simulink model "EcuAppM_StateMachine"  (R2022b)
settings: Solver=FixedStepDiscrete  StartTime=0  StopTime=50  FixedStep=1  RelTol=1e-3  EnableMultiTasking=on
values from neighbouring files (symbols this model uses):
  ECUAPPM_MAX_WAKEUP_SOURCES = mpt.Parameter    [EcuAppM_StateMachine_Param.m]    (also in EcuAppM_StateMachine_Param_For_Safety_Context.m)
  ECUAPPM_VALUE_ZERO = mpt.Parameter    [EcuAppM_StateMachine_Param.m]    (also in EcuAppM_StateMachine_Param_For_Safety_Context.m)
  EcuAppM_WakeupSourcesData = mpt.Parameter    [EcuAppM_StateMachine_Param.m]    (also in EcuAppM_StateMachine_Param_For_Safety_Context.m)
libraries: simulink x3
(part 1 of 2)
settings Model: Creator=CINISSAN  LastModifiedBy=akappa
settings SolverCC: AlgebraicLoopSolver=TrustRegion
settings DataIOCC: MaxDataPoints=1000000  SaveOutput=off  InspectSignalLogs=on  ReturnWorkspaceOutputs=off
settings OptimizationCC: DefaultParameterBehavior=Inlined  UseSpecifiedMinMax=on  PassReuseOutputArgsAs=Individual arguments  RollThreshold=2  ZeroExternalMemoryAtStartup=off  LifeSpan=1  MaxStackSize=750  OptimizationLevel=level1  EfficientTunableParamExpr=on
settings DebuggingCC: UnconnectedInputMsg=warning  UnconnectedOutputMsg=warning  UnconnectedLineMsg=warning  AllowSymbolicDim=off  SFUnexpectedBacktrackingDiag=warning  SFNoUnconditionalDefaultTransitionDiag=warning  SFExecutionAtInitializationDiag=none  SFMachineParentedDataDiag=warning  ArithmeticOperatorsInVariantConditions=warning
settings HardwareCC: ProdLongLongMode=on
settings ModelReferenceCC: EnableRefExpFcnMdlSchedulingChecks=on
settings SFSimCC: SimCustomHeaderCode="#include \"EcuAppMExt.h\""  SimUserSources=EcuAppMExt.c  SimUseLocalCustomCode=off  SimGenImportedTypeDefs=on  MATLABDynamicMemAlloc=off  CustomCodeUndefinedFunction=UseInterfaceOnly
settings RTWCC: Description=Embedded Coder  SystemTargetFile=ert.tlc  GenCodeOnly=on  TemplateMakefile=ert_default_tmf  GenerateReport=on  RetainRTWFile=on  RTWUseLocalCustomCode=off  CustomHeaderCode="#include \"EcuAppM_CmdProcessing.h\""  IncludeHyperlinkInReport=on  LaunchReport=on  PortableWordSizes=on  GenerateTraceInfo=on  GenerateTraceReport=on  GenerateTraceReportSl=on  GenerateTraceReportSf=on  GenerateTraceReportEml=on  GenerateCodeReplacementReport=on
settings CodeAppCC: IgnoreCustomStorageClasses=off  MaxIdLength=250  SimulinkBlockComments=off
settings ERTTargetCC: MultiwordLength=2048  GenerateSampleERTMain=on  SuppressErrorStatus=on  ParenthesesLevel=Maximum  CastingMode=Standards  InlinedParameterPlacement=NonHierarchical  ERTCustomFileTemplate=example_file_process.tlc  ERTFilePackagingFormat=CompactWithDataFile
settings ConfigComp: CovEnable=on  RecordCoverage=on  CovMetricSettings=dcmtw  CovHTMLOptions=-sRT=1 -sVT=0 -aTS=1 -agT=1 -bRG=1 -bTC=1 -hTR=0 -nFC=0 -nFD=1 -scm=1 -bcm=1 -xEv=1 -xEM=1 -req=1  CovSaveCumulativeToWorkspaceVar=on  CovCumulativeReport=on  CovModelRefEnable=on

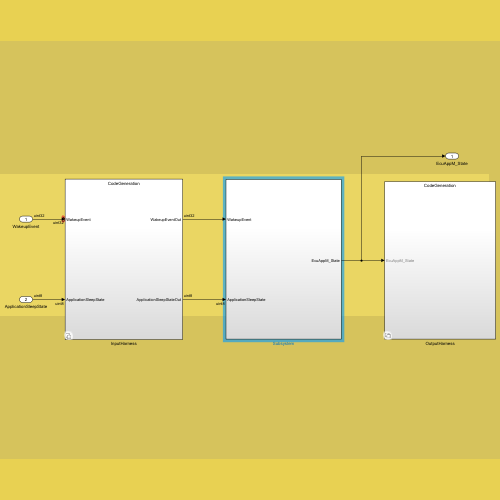
[thumbnail: Simulink's stored preview of the top-level diagram]
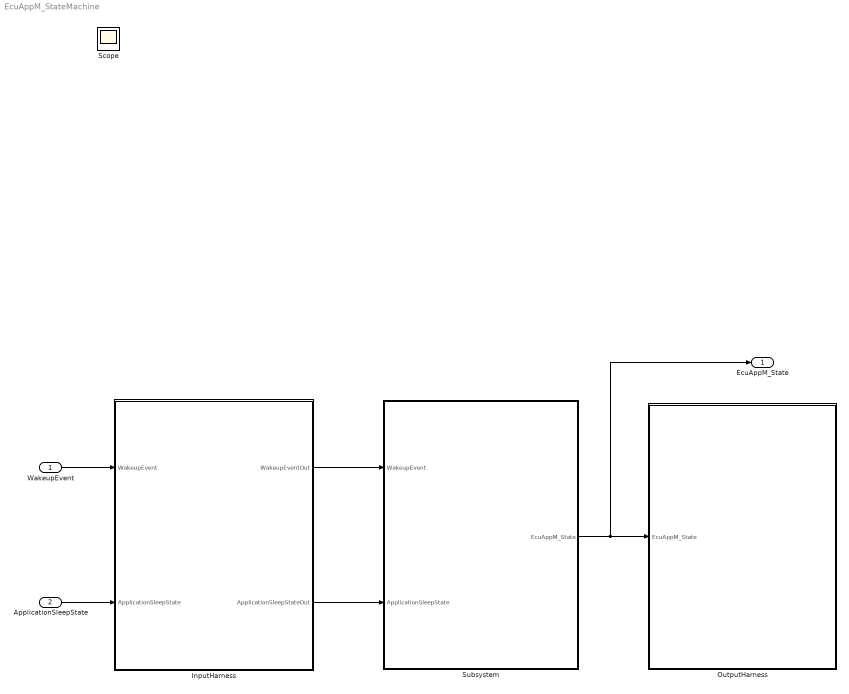
== system EcuAppM_StateMachine ==
  WakeupEvent : Inport  OutDataTypeStr=uint32
  ApplicationSleepState : Inport  Port=2  OutDataTypeStr=uint8
  InputHarness : Subsystem  Variant=on
  OutputHarness : Subsystem  Variant=on
  Subsystem : Subsystem
  EcuAppM_State : Outport  VectorParamsAs1DForOutWhenUnconnected=off
  Scope : Scope
  wires:
  ApplicationSleepState/1 -> InputHarness/2(ApplicationSleepState)
  InputHarness/1(WakeupEventOut) -> Subsystem/1(WakeupEvent)
  InputHarness/2(ApplicationSleepStateOut) -> Subsystem/2(ApplicationSleepState)
  Subsystem/1(EcuAppM_State) -> EcuAppM_State/1, OutputHarness/1(EcuAppM_State)
  WakeupEvent/1 -> InputHarness/1(WakeupEvent)

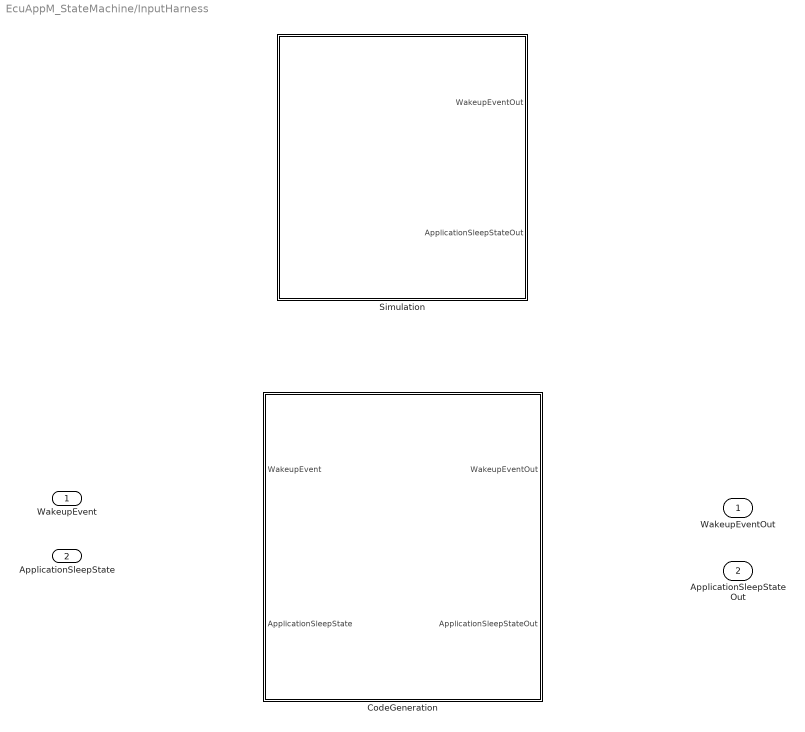
== system EcuAppM_StateMachine/InputHarness ==
  WakeupEvent : Inport  OutDataTypeStr=uint32
  ApplicationSleepState : Inport  Port=2  OutDataTypeStr=uint8
  CodeGeneration : Subsystem  VariantControl=CODEGENERATION
  Simulation : Subsystem  VariantControl=SIMULATION
  WakeupEventOut : Outport  OutDataTypeStr=uint32  PortDimensions=1  VectorParamsAs1DForOutWhenUnconnected=off
  ApplicationSleepStateOut : Outport  Port=2  OutDataTypeStr=uint8  PortDimensions=1  VectorParamsAs1DForOutWhenUnconnected=off

== system EcuAppM_StateMachine/OutputHarness ==
  EcuAppM_State : Inport
  CodeGeneration : Subsystem  VariantControl=CODEGENERATION
  Simulation : Subsystem  VariantControl=SIMULATION

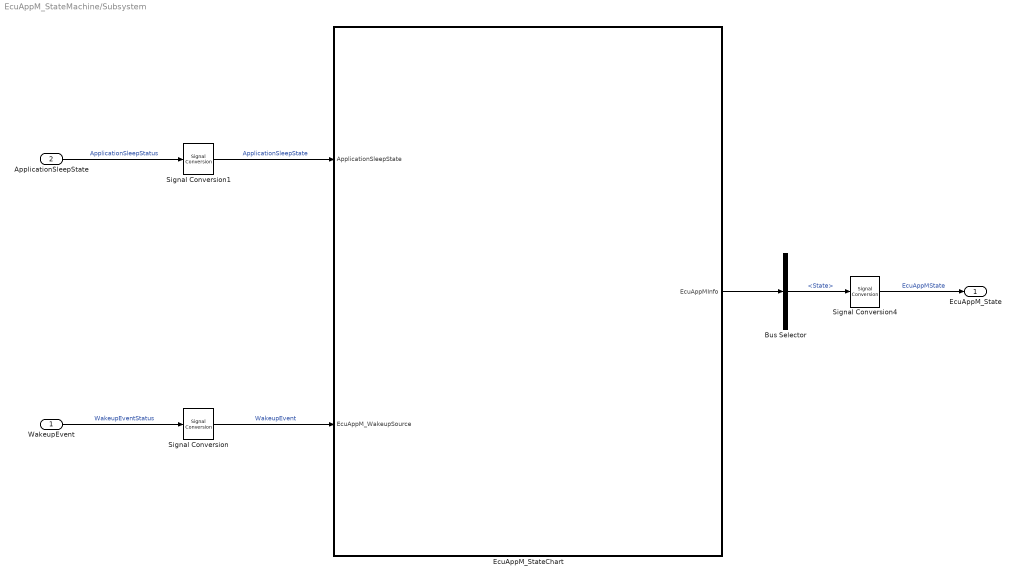
== system EcuAppM_StateMachine/Subsystem ==
  WakeupEvent : Inport  OutDataTypeStr=uint32
  ApplicationSleepState : Inport  Port=2  OutDataTypeStr=uint8
  Bus Selector : BusSelector  OutputSignals=State
  EcuAppM_StateChart : Stateflow chart  TreatAsAtomicUnit=on  RTWFcnName=EcuAppM_StateChart
      settings: RTWSystemCode=Nonreusable function  RTWFcnNameOpts=User specified
  Signal Conversion : SignalConversion  OverrideOpt=off
  Signal Conversion1 : SignalConversion  OverrideOpt=off
  Signal Conversion4 : SignalConversion  OverrideOpt=off
  EcuAppM_State : Outport  PortDimensions=1  VectorParamsAs1DForOutWhenUnconnected=off
  wires:
  WakeupEvent/1 -> Signal Conversion/1  "WakeupEventStatus"
  ApplicationSleepState/1 -> Signal Conversion1/1  "ApplicationSleepStatus"
  Signal Conversion1/1 -> EcuAppM_StateChart/1(ApplicationSleepState)  "ApplicationSleepState"
  Signal Conversion/1 -> EcuAppM_StateChart/2(EcuAppM_WakeupSource)  "WakeupEvent"
  EcuAppM_StateChart/1(EcuAppMInfo) -> Bus Selector/1
  Bus Selector/1 -> Signal Conversion4/1  "<State>"
  Signal Conversion4/1 -> EcuAppM_State/1  "EcuAppMState"

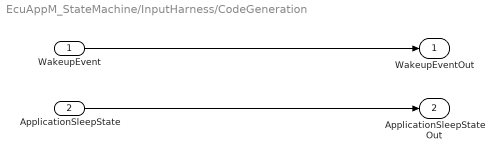
== system EcuAppM_StateMachine/InputHarness/CodeGeneration ==
  WakeupEvent : Inport
  ApplicationSleepState : Inport  Port=2  OutDataTypeStr=uint8
  WakeupEventOut : Outport  OutDataTypeStr=uint32  PortDimensions=1  VectorParamsAs1DForOutWhenUnconnected=off
  ApplicationSleepStateOut : Outport  Port=2  OutDataTypeStr=uint8  PortDimensions=1  VectorParamsAs1DForOutWhenUnconnected=off
  wires:
  WakeupEvent/1 -> WakeupEventOut/1
  ApplicationSleepState/1 -> ApplicationSleepStateOut/1

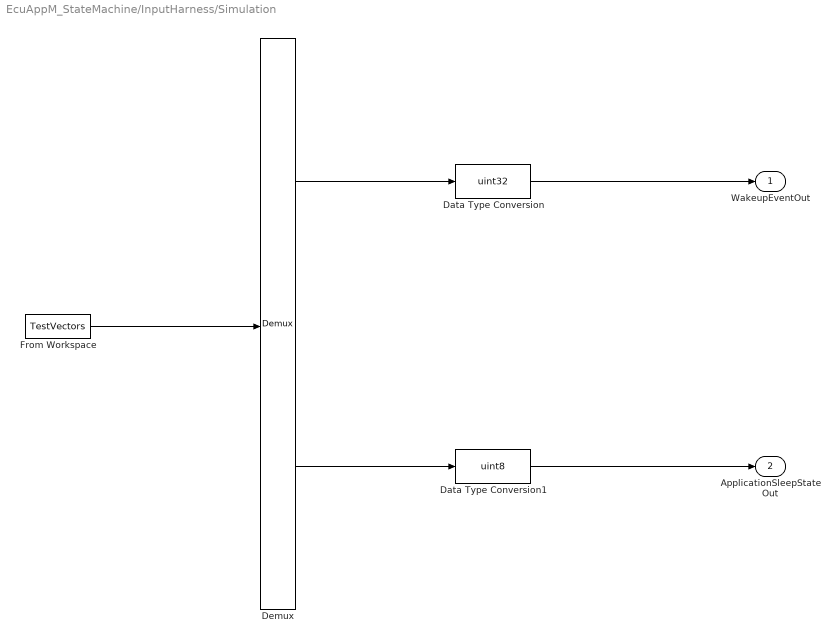
== system EcuAppM_StateMachine/InputHarness/Simulation ==
  Data Type Conversion : DataTypeConversion  OutDataTypeStr=uint32  SaturateOnIntegerOverflow=off  RndMeth=Floor
  Data Type Conversion1 : DataTypeConversion  OutDataTypeStr=uint8  SaturateOnIntegerOverflow=off  RndMeth=Floor
  Demux : Demux  Outputs=2
  From Workspace : FromWorkspace  VariableName=TestVectors  SampleTime=1  Interpolate=off  OutputAfterFinalValue=Holding final value
  WakeupEventOut : Outport  OutDataTypeStr=uint32  PortDimensions=1  VectorParamsAs1DForOutWhenUnconnected=off
  ApplicationSleepStateOut : Outport  Port=2  OutDataTypeStr=uint8  PortDimensions=1  VectorParamsAs1DForOutWhenUnconnected=off
  wires:
  Demux/1 -> Data Type Conversion/1
  Demux/2 -> Data Type Conversion1/1
  From Workspace/1 -> Demux/1
  Data Type Conversion/1 -> WakeupEventOut/1
  Data Type Conversion1/1 -> ApplicationSleepStateOut/1

== system EcuAppM_StateMachine/OutputHarness/CodeGeneration ==

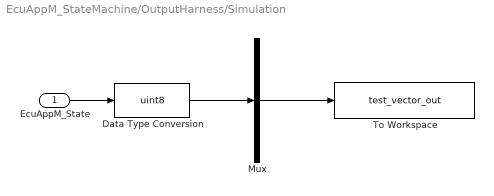
== system EcuAppM_StateMachine/OutputHarness/Simulation ==
  EcuAppM_State : Inport
  Data Type Conversion : DataTypeConversion  OutDataTypeStr=uint8  SaturateOnIntegerOverflow=off  RndMeth=Floor
  Mux : Mux  Inputs=1
  To Workspace : ToWorkspace  VariableName=test_vector_out  SampleTime=1
      settings: Save2DSignal=2-D array (concatenate along first dimension)
  wires:
  EcuAppM_State/1 -> Data Type Conversion/1
  Mux/1 -> To Workspace/1
  Data Type Conversion/1 -> Mux/1

== system EcuAppM_StateMachine/Subsystem/EcuAppM_StateChart/EcuAppM_BackupDataWrapper ==
  f : TriggerPort  TriggerType=function-call  VariantControl=(inherit)
      settings: CopyFcn=Stateflow.SLINSF.SimulinkMan.removeBlockPreDeleteFcn  PreDeleteFcn=Stateflow.SLINSF.SimulinkMan.unsafePredeleteFcn
  C Caller : CCaller  FunctionName=EcuAppM_BackupData

== system EcuAppM_StateMachine/Subsystem/EcuAppM_StateChart/EcuAppM_ClearWakeupReasonWrapper ==
  f : TriggerPort  TriggerType=function-call  VariantControl=(inherit)
      settings: CopyFcn=Stateflow.SLINSF.SimulinkMan.removeBlockPreDeleteFcn  PreDeleteFcn=Stateflow.SLINSF.SimulinkMan.unsafePredeleteFcn
  C Caller : CCaller  FunctionName=EcuAppM_ClearWakeupSources

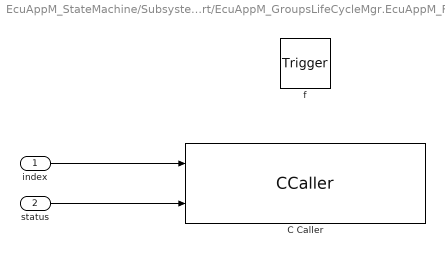
== system EcuAppM_StateMachine/Subsystem/EcuAppM_StateChart/EcuAppM_GroupsLifeCycleMgr.EcuAppM_FailSafeMechanismWrapper ==
  index : Inport  OutDataTypeStr=uint8  PortDimensions=1
  status : Inport  Port=2  OutDataTypeStr=uint8  PortDimensions=1
  f : TriggerPort  TriggerType=function-call  VariantControl=(inherit)
      settings: CopyFcn=Stateflow.SLINSF.SimulinkMan.removeBlockPreDeleteFcn  PreDeleteFcn=Stateflow.SLINSF.SimulinkMan.unsafePredeleteFcn
  C Caller : CCaller  FunctionName=EcuAppM_FailSafeMechanism  PortSpecificationStruct="%)30     .    V ,   8    (     @         %    \"     (    !     0         %  0 \"0    $    _    07)G3F%M90  4&]R=$YA;64 4V-O<&4     26YD97@     5'EP90      4VEZ90      27-';&]B86P   X    X    !@    @    $          4    (     0    <    !         !     '    1W)O=7!)9  .    .     8    (    !          %    \"     $    '     0         0    !P   $=R;W5P260 #@   #@    &    \"     0         !0    @    !    !0    $         $     4   !);G!U=     X    X    !@    @    &          4    (     0    $    !          D    (               .    .     8    (    !          %    \"     $    %     0         0    !0   '5I;G0X    #@   #     &    \"     0         !0    @    !     0    $         $  ! #$    .    ,     8    (    \"0(        %    \"     $    !     0         \"  $       X    X    !@    @    $          4    (     0    4    !         !     %    4W1A=&4    .    .     8    (    !          %    \"     $    %     0         0    !0   %-T871E    #@   #@    &    \"     0         !0    @    !    !0    $         $     4   !);G!U=     X    X    !@    @    &          4    (     0    $    !          D    (            \\#\\.    .     8    (    !          %    \"     $    %     0         0    !0   '5I;G0X    #@   #     &    \"     0         !0    @    !     0    $         $  ! #$    .    ,     8    (    \"0(        %    \"     $    !     0         \"  $"
  wires:
  index/1 -> C Caller/1
  status/1 -> C Caller/2

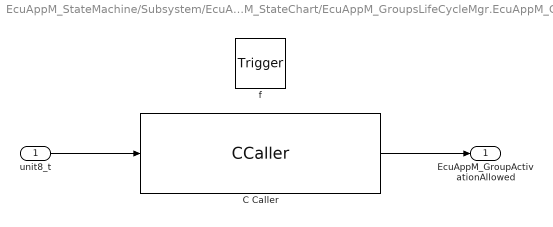
== system EcuAppM_StateMachine/Subsystem/EcuAppM_StateChart/EcuAppM_GroupsLifeCycleMgr.EcuAppM_GroupActivationCalloutWrapper ==
  unit8_t : Inport  OutDataTypeStr=uint8  PortDimensions=1  LockScale=on
  f : TriggerPort  TriggerType=function-call  VariantControl=(inherit)
      settings: CopyFcn=Stateflow.SLINSF.SimulinkMan.removeBlockPreDeleteFcn  PreDeleteFcn=Stateflow.SLINSF.SimulinkMan.unsafePredeleteFcn
  C Caller : CCaller  FunctionName=EcuAppM_GroupActivationCallout  PortSpecificationStruct="%)30     .    R ,   8    (     @         %    \"     (    !     0         %  0 \"0    $    _    07)G3F%M90  4&]R=$YA;64 4V-O<&4     26YD97@     5'EP90      4VEZ90      27-';&]B86P   X    P    !@    @    $          4    (     0    ,    !         !   P!O=70 #@   #     &    \"     0         !0    @    !     P    $         $  # &]U=  .    .     8    (    !          %    \"     $    &     0         0    !@   $]U='!U=   #@   #@    &    \"     8         !0    @    !     0    $         \"0    @               X    X    !@    @    $          4    (     0    4    !         !     %    =6EN=#@    .    ,     8    (    !          %    \"     $    !     0         0  $ ,0    X    P    !@    @    ) @        4    (     0    $    !          (  0      #@   #@    &    \"     0         !0    @    !    !P    $         $     <   !'<F]U<$ED  X    X    !@    @    $          4    (     0    <    !         !     '    1W)O=7!)9  .    .     8    (    !          %    \"     $    %     0         0    !0   $EN<'5T    #@   #@    &    \"     8         !0    @    !     0    $         \"0    @               X    X    !@    @    $          4    (     0    4    !         !     %    =6EN=#@    .    ,     8    (    !          %    \"     $    !     0         0  $ ,0    X    P    !@    @    ) @        4    (     0    $    !          (  0"
  EcuAppM_GroupActivationAllowed : Outport
  wires:
  unit8_t/1 -> C Caller/1
  C Caller/1 -> EcuAppM_GroupActivationAllowed/1

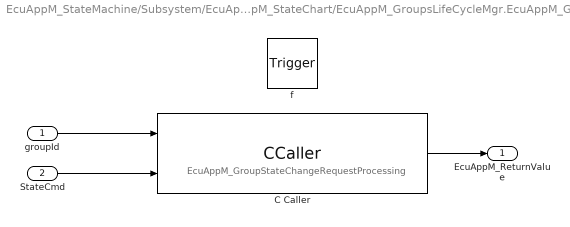
== system EcuAppM_StateMachine/Subsystem/EcuAppM_StateChart/EcuAppM_GroupsLifeCycleMgr.EcuAppM_GroupStateChangeRequestWrapper ==
  note: EcuAppM_GroupStateChangeRequestProcessing
  groupId : Inport  OutDataTypeStr=uint8  PortDimensions=1  LockScale=on
  StateCmd : Inport  Port=2  OutDataTypeStr=uint8  PortDimensions=1
  f : TriggerPort  TriggerType=function-call  VariantControl=(inherit)
      settings: CopyFcn=Stateflow.SLINSF.SimulinkMan.removeBlockPreDeleteFcn  PreDeleteFcn=Stateflow.SLINSF.SimulinkMan.unsafePredeleteFcn
  C Caller : CCaller  FunctionName=EcuAppM_GroupStateChangeRequestProcessing  PortSpecificationStruct="%)30     .    B 4   8    (     @         %    \"     ,    !     0         %  0 \"0    $    _    07)G3F%M90  4&]R=$YA;64 4V-O<&4     26YD97@     5'EP90      4VEZ90      27-';&]B86P   X    P    !@    @    $          4    (     0    ,    !         !   P!O=70 #@   #     &    \"     0         !0    @    !     P    $         $  # &]U=  .    .     8    (    !          %    \"     $    &     0         0    !@   $]U='!U=   #@   #@    &    \"     8         !0    @    !     0    $         \"0    @               X    X    !@    @    $          4    (     0    4    !         !     %    =6EN=#@    .    ,     8    (    !          %    \"     $    !     0         0  $ ,0    X    P    !@    @    ) @        4    (     0    $    !          (  0      #@   #@    &    \"     0         !0    @    !    !P    $         $     <   !G<F]U<$ED  X    X    !@    @    $          4    (     0    <    !         !     '    9W)O=7!)9  .    .     8    (    !          %    \"     $    %     0         0    !0   $EN<'5T    #@   #@    &    \"     8         !0    @    !     0    $         \"0    @               X    X    !@    @    $          4    (     0    4    !         !     %    =6EN=#@    .    ,     8    (    !          %    \"     $    !     0         0  $ ,0    X    P    !@    @    ) @        4    (     0    $    !          (  0      #@   $     &    \"     0         !0    @    !    \"@    $         $     H   !G<F]U<%-T871E        #@   $     &    \"     0         !0    @    !    \"@    $         $     H   !G<F]U<%-T871E        #@   #@    &    \"     0         !0    @    !    !0    $         $     4   !);G!U=     X    X    !@    @    &          4    (     0    $    !          D    (            \\#\\.    .     8    (    !          %    \"     $    %     0         0    !0   '5I;G0X    #@   #     &    \"     0         !0    @    !     0    $         $  ! #$    .    ,     8    (    \"0(        %    \"     $    !     0         \"  $"
  EcuAppM_ReturnValue : Outport
  wires:
  groupId/1 -> C Caller/1
  C Caller/1 -> EcuAppM_ReturnValue/1
  StateCmd/1 -> C Caller/2

== system EcuAppM_StateMachine/Subsystem/EcuAppM_StateChart/EcuAppM_GroupsLifeCycleMgr.EcuAppM_GroupStatusChangeCbkWrapper ==
  index : Inport  OutDataTypeStr=uint8  PortDimensions=1
  status : Inport  Port=2  OutDataTypeStr=uint8  PortDimensions=1
  f : TriggerPort  TriggerType=function-call  VariantControl=(inherit)
      settings: CopyFcn=Stateflow.SLINSF.SimulinkMan.removeBlockPreDeleteFcn  PreDeleteFcn=Stateflow.SLINSF.SimulinkMan.unsafePredeleteFcn
  C Caller : CCaller  FunctionName=EcuAppM_GroupStatusChangeCbk  PortSpecificationStruct="%)30     .    Z ,   8    (     @         %    \"     (    !     0         %  0 \"0    $    _    07)G3F%M90  4&]R=$YA;64 4V-O<&4     26YD97@     5'EP90      4VEZ90      27-';&]B86P   X    X    !@    @    $          4    (     0    <    !         !     '    9W)O=7!)9  .    .     8    (    !          %    \"     $    '     0         0    !P   &=R;W5P260 #@   #@    &    \"     0         !0    @    !    !0    $         $     4   !);G!U=     X    X    !@    @    &          4    (     0    $    !          D    (               .    .     8    (    !          %    \"     $    %     0         0    !0   '5I;G0X    #@   #     &    \"     0         !0    @    !     0    $         $  ! #$    .    ,     8    (    \"0(        %    \"     $    !     0         \"  $       X   !     !@    @    $          4    (     0    H    !         !     *    9W)O=7!3=&%T90        X   !     !@    @    $          4    (     0    H    !         !     *    9W)O=7!3=&%T90        X    X    !@    @    $          4    (     0    4    !         !     %    26YP=70    .    .     8    (    !@         %    \"     $    !     0         )    \"            / _#@   #@    &    \"     0         !0    @    !    !0    $         $     4   !U:6YT.     X    P    !@    @    $          4    (     0    $    !         !   0 Q    #@   #     &    \"     D\"        !0    @    !     0    $          @ !"
  wires:
  index/1 -> C Caller/1
  status/1 -> C Caller/2

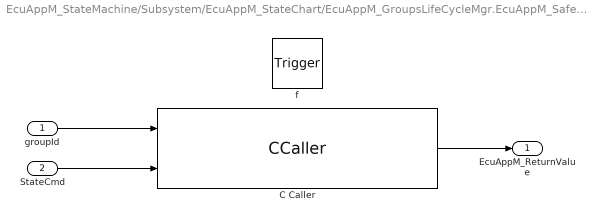
== system EcuAppM_StateMachine/Subsystem/EcuAppM_StateChart/EcuAppM_GroupsLifeCycleMgr.EcuAppM_SafeGroupStateChangeRequestWrapper ==
  groupId : Inport  OutDataTypeStr=uint8  PortDimensions=1  LockScale=on
  StateCmd : Inport  Port=2  OutDataTypeStr=uint8  PortDimensions=1
  f : TriggerPort  TriggerType=function-call  VariantControl=(inherit)
      settings: CopyFcn=Stateflow.SLINSF.SimulinkMan.removeBlockPreDeleteFcn  PreDeleteFcn=Stateflow.SLINSF.SimulinkMan.unsafePredeleteFcn
  C Caller : CCaller  FunctionName=EcuAppM_DispatchSafeGroupStateChangeRequest  PortSpecificationStruct="%)30     .    B 4   8    (     @         %    \"     ,    !     0         %  0 \"0    $    _    07)G3F%M90  4&]R=$YA;64 4V-O<&4     26YD97@     5'EP90      4VEZ90      27-';&]B86P   X    P    !@    @    $          4    (     0    ,    !         !   P!O=70 #@   #     &    \"     0         !0    @    !     P    $         $  # &]U=  .    .     8    (    !          %    \"     $    &     0         0    !@   $]U='!U=   #@   #@    &    \"     8         !0    @    !     0    $         \"0    @               X    X    !@    @    $          4    (     0    4    !         !     %    =6EN=#@    .    ,     8    (    !          %    \"     $    !     0         0  $ ,0    X    P    !@    @    ) @        4    (     0    $    !          (  0      #@   #@    &    \"     0         !0    @    !    !P    $         $     <   !G<F]U<$ED  X    X    !@    @    $          4    (     0    <    !         !     '    9W)O=7!)9  .    .     8    (    !          %    \"     $    %     0         0    !0   $EN<'5T    #@   #@    &    \"     8         !0    @    !     0    $         \"0    @               X    X    !@    @    $          4    (     0    4    !         !     %    =6EN=#@    .    ,     8    (    !          %    \"     $    !     0         0  $ ,0    X    P    !@    @    ) @        4    (     0    $    !          (  0      #@   $     &    \"     0         !0    @    !    \"@    $         $     H   !G<F]U<%-T871E        #@   $     &    \"     0         !0    @    !    \"@    $         $     H   !G<F]U<%-T871E        #@   #@    &    \"     0         !0    @    !    !0    $         $     4   !);G!U=     X    X    !@    @    &          4    (     0    $    !          D    (            \\#\\.    .     8    (    !          %    \"     $    %     0         0    !0   '5I;G0X    #@   #     &    \"     0         !0    @    !     0    $         $  ! #$    .    ,     8    (    \"0(        %    \"     $    !     0         \"  $"
  EcuAppM_ReturnValue : Outport
  wires:
  groupId/1 -> C Caller/1
  StateCmd/1 -> C Caller/2
  C Caller/1 -> EcuAppM_ReturnValue/1

== system EcuAppM_StateMachine/Subsystem/EcuAppM_StateChart/EcuAppM_OnNVMReadAllWrapper ==
  EcuAppM_BufferedWakeupSource : Inport  OutDataTypeStr=uint32  PortDimensions=1
  f : TriggerPort  TriggerType=function-call  VariantControl=(inherit)
      settings: CopyFcn=Stateflow.SLINSF.SimulinkMan.removeBlockPreDeleteFcn  PreDeleteFcn=Stateflow.SLINSF.SimulinkMan.unsafePredeleteFcn
  C Caller : CCaller  FunctionName=EcuAppM_OnNVMReadAll  PortSpecificationStruct="%)30     .    . (   8    (     @         %    \"     $    !     0         %  0 \"0    $    _    07)G3F%M90  4&]R=$YA;64 4V-O<&4     26YD97@     5'EP90      4VEZ90      27-';&]B86P   X   !     !@    @    $          4    (     0    P    !         !     ,    5V%K975P4V]U<F-E      X   !     !@    @    $          4    (     0    P    !         !     ,    5V%K975P4V]U<F-E      X    X    !@    @    $          4    (     0    4    !         !     %    26YP=70    .    .     8    (    !@         %    \"     $    !     0         )    \"               #@   #@    &    \"     0         !0    @    !    !@    $         $     8   !U:6YT,38   X    P    !@    @    $          4    (     0    $    !         !   0 Q    #@   #     &    \"     D\"        !0    @    !     0    $          @ !"
  wires:
  EcuAppM_BufferedWakeupSource/1 -> C Caller/1

== system EcuAppM_StateMachine/Subsystem/EcuAppM_StateChart/EcuAppM_OnPowerSeqStartWrapper ==
  State : Inport  OutDataTypeStr=uint8  PortDimensions=1  LockScale=on
  f : TriggerPort  TriggerType=function-call  VariantControl=(inherit)
      settings: CopyFcn=Stateflow.SLINSF.SimulinkMan.removeBlockPreDeleteFcn  PreDeleteFcn=Stateflow.SLINSF.SimulinkMan.unsafePredeleteFcn
  C Caller : CCaller  FunctionName=EcuAppM_OnPowerSeqStart  PortSpecificationStruct="%)30     .    * (   8    (     @         %    \"     $    !     0         %  0 \"0    $    _    07)G3F%M90  4&]R=$YA;64 4V-O<&4     26YD97@     5'EP90      4VEZ90      27-';&]B86P   X    X    !@    @    $          4    (     0    4    !         !     %    4W1A=&4    .    .     8    (    !          %    \"     $    %     0         0    !0   %-T871E    #@   #@    &    \"     0         !0    @    !    !0    $         $     4   !);G!U=     X    X    !@    @    &          4    (     0    $    !          D    (               .    .     8    (    !          %    \"     $    %     0         0    !0   '5I;G0X    #@   #     &    \"     0         !0    @    !     0    $         $  ! #$    .    ,     8    (    \"0(        %    \"     $    !     0         \"  $"
  wires:
  State/1 -> C Caller/1

== system EcuAppM_StateMachine/Subsystem/EcuAppM_StateChart/EcuAppM_OnStartupWrapper ==
  EcuAppM_BufferedWakeupSource : Inport  OutDataTypeStr=uint32  PortDimensions=1
  f : TriggerPort  TriggerType=function-call  VariantControl=(inherit)
      settings: CopyFcn=Stateflow.SLINSF.SimulinkMan.removeBlockPreDeleteFcn  PreDeleteFcn=Stateflow.SLINSF.SimulinkMan.unsafePredeleteFcn
  C Caller : CCaller  FunctionName=EcuAppM_OnStartup  PortSpecificationStruct="%)30     .    . (   8    (     @         %    \"     $    !     0         %  0 \"0    $    _    07)G3F%M90  4&]R=$YA;64 4V-O<&4     26YD97@     5'EP90      4VEZ90      27-';&]B86P   X   !     !@    @    $          4    (     0    P    !         !     ,    5V%K975P4V]U<F-E      X   !     !@    @    $          4    (     0    P    !         !     ,    5V%K975P4V]U<F-E      X    X    !@    @    $          4    (     0    4    !         !     %    26YP=70    .    .     8    (    !@         %    \"     $    !     0         )    \"               #@   #@    &    \"     0         !0    @    !    !@    $         $     8   !U:6YT,S(   X    P    !@    @    $          4    (     0    $    !         !   0 Q    #@   #     &    \"     D\"        !0    @    !     0    $          @ !"
  wires:
  EcuAppM_BufferedWakeupSource/1 -> C Caller/1

== system EcuAppM_StateMachine/Subsystem/EcuAppM_StateChart/EcuAppM_OnWakeupValidationWrapper ==
  EcuAppM_BufferedWakeupSource : Inport  OutDataTypeStr=uint32  PortDimensions=1
  f : TriggerPort  TriggerType=function-call  VariantControl=(inherit)
      settings: CopyFcn=Stateflow.SLINSF.SimulinkMan.removeBlockPreDeleteFcn  PreDeleteFcn=Stateflow.SLINSF.SimulinkMan.unsafePredeleteFcn
  C Caller : CCaller  FunctionName=EcuAppM_OnWakeupValidation  PortSpecificationStruct="%)30     .    . (   8    (     @         %    \"     $    !     0         %  0 \"0    $    _    07)G3F%M90  4&]R=$YA;64 4V-O<&4     26YD97@     5'EP90      4VEZ90      27-';&]B86P   X   !     !@    @    $          4    (     0    P    !         !     ,    5V%K975P4V]U<F-E      X   !     !@    @    $          4    (     0    P    !         !     ,    5V%K975P4V]U<F-E      X    X    !@    @    $          4    (     0    4    !         !     %    26YP=70    .    .     8    (    !@         %    \"     $    !     0         )    \"               #@   #@    &    \"     0         !0    @    !    !@    $         $     8   !U:6YT,S(   X    P    !@    @    $          4    (     0    $    !         !   0 Q    #@   #     &    \"     D\"        !0    @    !     0    $          @ !"
  wires:
  EcuAppM_BufferedWakeupSource/1 -> C Caller/1

== system EcuAppM_StateMachine/Subsystem/EcuAppM_StateChart/EcuAppM_ProcessJobStatusWrapper.EcuAppM_ProcessJobStatusFunc ==
  state : Inport  OutDataTypeStr=uint8  PortDimensions=1
  f : TriggerPort  TriggerType=function-call  VariantControl=(inherit)
      settings: CopyFcn=Stateflow.SLINSF.SimulinkMan.removeBlockPreDeleteFcn  PreDeleteFcn=Stateflow.SLINSF.SimulinkMan.unsafePredeleteFcn
  C Caller : CCaller  FunctionName=EcuAppM_ProcessJobStatus  PortSpecificationStruct="%)30     .    R ,   8    (     @         %    \"     (    !     0         %  0 \"0    $    _    07)G3F%M90  4&]R=$YA;64 4V-O<&4     26YD97@     5'EP90      4VEZ90      27-';&]B86P   X    P    !@    @    $          4    (     0    ,    !         !   P!O=70 #@   #     &    \"     0         !0    @    !     P    $         $  # &]U=  .    .     8    (    !          %    \"     $    &     0         0    !@   $]U='!U=   #@   #@    &    \"     8         !0    @    !     0    $         \"0    @               X    X    !@    @    $          4    (     0    4    !         !     %    =6EN=#@    .    ,     8    (    !          %    \"     $    !     0         0  $ ,0    X    P    !@    @    ) @        4    (     0    $    !          (  0      #@   #@    &    \"     0         !0    @    !    !0    $         $     4   !S=&%T90    X    X    !@    @    $          4    (     0    4    !         !     %    <W1A=&4    .    .     8    (    !          %    \"     $    %     0         0    !0   $EN<'5T    #@   #@    &    \"     8         !0    @    !     0    $         \"0    @               X    X    !@    @    $          4    (     0    4    !         !     %    =6EN=#@    .    ,     8    (    !          %    \"     $    !     0         0  $ ,0    X    P    !@    @    ) @        4    (     0    $    !          (  0"
  status : Outport  OutDataTypeStr=uint8  PortDimensions=1
  wires:
  state/1 -> C Caller/1
  C Caller/1 -> status/1

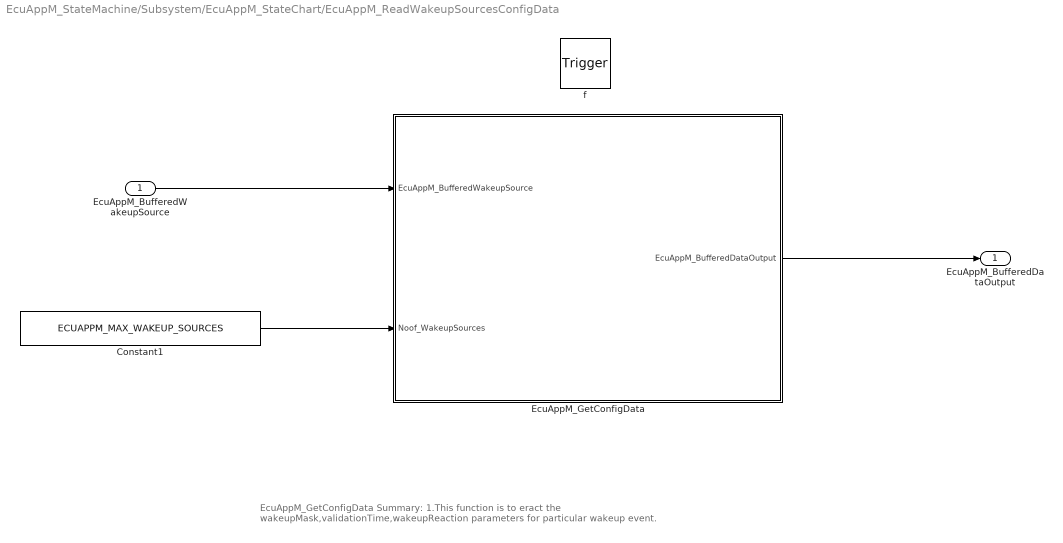
== system EcuAppM_StateMachine/Subsystem/EcuAppM_StateChart/EcuAppM_ReadWakeupSourcesConfigData ==
  note: EcuAppM_GetConfigData Summary:
      |
      | 1.This function is to eract the wakeupMask,validationTime,wakeupReaction parameters for particular wakeup event.
  EcuAppM_BufferedWakeupSource : Inport  OutDataTypeStr=uint32  PortDimensions=1
  f : TriggerPort  TriggerType=function-call  VariantControl=(inherit)
      settings: CopyFcn=Stateflow.SLINSF.SimulinkMan.removeBlockPreDeleteFcn  PreDeleteFcn=Stateflow.SLINSF.SimulinkMan.unsafePredeleteFcn
  Constant1 : Constant  Value=ECUAPPM_MAX_WAKEUP_SOURCES  OutDataTypeStr=uint16  SampleTime=-1
  EcuAppM_GetConfigData : Subsystem  TreatAsAtomicUnit=on  RTWFcnName=EcuAppM_GetConfigData
      settings: RTWFcnNameOpts=User specified
  EcuAppM_BufferedDataOutput : Outport  OutDataTypeStr=Bus: EcuAppM_WakeupSourcesType  PortDimensions=1  InitialOutput=[0]
  wires:
  EcuAppM_BufferedWakeupSource/1 -> EcuAppM_GetConfigData/1(EcuAppM_BufferedWakeupSource)
  Constant1/1 -> EcuAppM_GetConfigData/2(Noof_WakeupSources)
  EcuAppM_GetConfigData/1(EcuAppM_BufferedDataOutput) -> EcuAppM_BufferedDataOutput/1

== system EcuAppM_StateMachine/Subsystem/EcuAppM_StateChart/EcuAppM_StartOfGroupsDeactivationWrapper ==
  f : TriggerPort  TriggerType=function-call  VariantControl=(inherit)
      settings: CopyFcn=Stateflow.SLINSF.SimulinkMan.removeBlockPreDeleteFcn  PreDeleteFcn=Stateflow.SLINSF.SimulinkMan.unsafePredeleteFcn
  C Caller : CCaller  FunctionName=EcuAppM_StartOfGroupsDeactivation

== system EcuAppM_StateMachine/Subsystem/EcuAppM_StateChart/EcuAppM_StartOfSleepTransientWrapper ==
  f : TriggerPort  TriggerType=function-call  VariantControl=(inherit)
      settings: CopyFcn=Stateflow.SLINSF.SimulinkMan.removeBlockPreDeleteFcn  PreDeleteFcn=Stateflow.SLINSF.SimulinkMan.unsafePredeleteFcn
  C Caller : CCaller  FunctionName=EcuAppM_StartOfSleepTransient

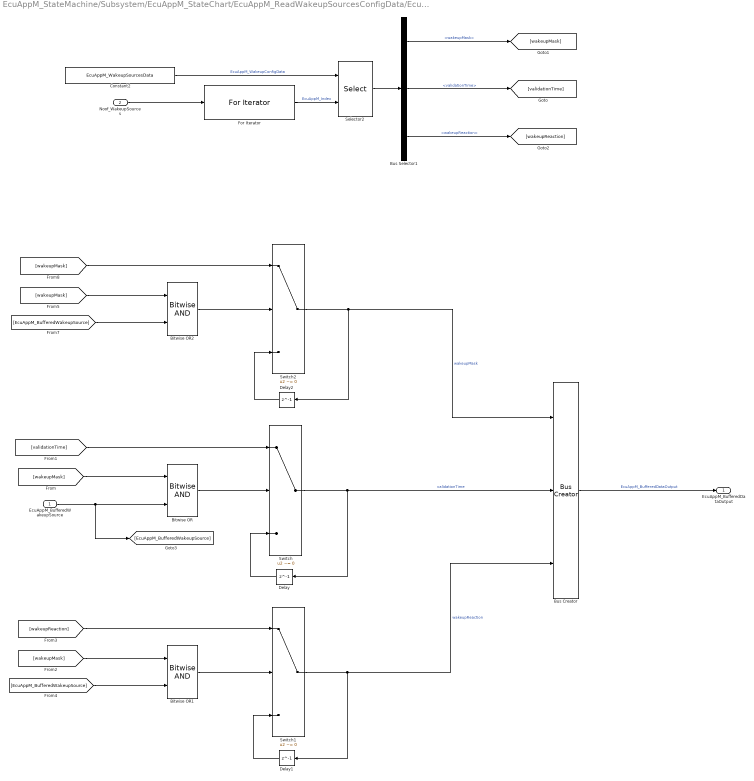
== system EcuAppM_StateMachine/Subsystem/EcuAppM_StateChart/EcuAppM_ReadWakeupSourcesConfigData/EcuAppM_GetConfigData ==
  EcuAppM_BufferedWakeupSource : Inport  PortDimensions=1
  Noof_WakeupSources : Inport  Port=2
  Bitwise OR : simulink/Logic and Bit Operations/Bitwise Operator  logicop=AND  UseBitMask=off  NumInputPorts=2  BitMask=bin2dec('11011001')  BitMaskRealWorld=Stored Integer
      settings: LibrarySourceBlock=|
      | simulink/Quick Insert/Logic and Bit
      | Operations/Bitwise OR
  Bitwise OR1 : simulink/Logic and Bit Operations/Bitwise Operator  logicop=AND  UseBitMask=off  NumInputPorts=2  BitMask=bin2dec('11011001')  BitMaskRealWorld=Stored Integer
      settings: LibrarySourceBlock=|
      | simulink/Quick Insert/Logic and Bit
      | Operations/Bitwise OR
  Bitwise OR2 : simulink/Logic and Bit Operations/Bitwise Operator  logicop=AND  UseBitMask=off  NumInputPorts=2  BitMask=bin2dec('11011001')  BitMaskRealWorld=Stored Integer
      settings: LibrarySourceBlock=|
      | simulink/Quick Insert/Logic and Bit
      | Operations/Bitwise OR
  Bus Creator : BusCreator  Inputs=3  OutDataTypeStr=Bus: EcuAppM_WakeupSourcesType  NonVirtualBus=on
  Bus Selector1 : BusSelector  OutputSignals=wakeupMask,validationTime,wakeupReaction
  Constant2 : Constant  Value=EcuAppM_WakeupSourcesData  OutDataTypeStr=Bus: EcuAppM_WakeupSourcesType
  Delay : Delay  DelayLength=1  InitialCondition=ECUAPPM_VALUE_ZERO  StateName=PrevvalidationTime  StateMustResolveToSignalObject=on
  Delay1 : Delay  DelayLength=1  InitialCondition=ECUAPPM_VALUE_ZERO  StateName=PrevwakeupReaction  StateMustResolveToSignalObject=on
  Delay2 : Delay  DelayLength=1  InitialCondition=ECUAPPM_VALUE_ZERO  StateName=PrevwakeupMask  StateMustResolveToSignalObject=on
  For Iterator : ForIterator  IterationSource=external  IterationLimit=MAX_NO_OF_WAKEUPS  IndexMode=Zero-based  IterationVariableDataType=uint16
  Selector2 : Selector  IndexMode=Zero-based  IndexOptions=Index vector (port)  Indices=[1 3]  OutputSizes=1
  Switch : Switch  Criteria=u2 ~= 0  OutDataTypeStr=uint16  SaturateOnIntegerOverflow=off  InputSameDT=off
  Switch1 : Switch  Criteria=u2 ~= 0  OutDataTypeStr=uint16  SaturateOnIntegerOverflow=off  InputSameDT=off
  Switch2 : Switch  Criteria=u2 ~= 0  OutDataTypeStr=uint32  SaturateOnIntegerOverflow=off  InputSameDT=off
  EcuAppM_BufferedDataOutput : Outport
  wires:
  Constant2/1 -> Selector2/1  "EcuAppM_WakeupConfigData"
  For Iterator/1 -> Selector2/2  "EcuAppM_Index"
  Selector2/1 -> Bus Selector1/1
  Noof_WakeupSources/1 -> For Iterator/1
  Bus Selector1/2 -> [validationTime]  "<validationTime>"
  Bus Selector1/1 -> [wakeupMask]  "<wakeupMask>"
  [wakeupMask] -> Bitwise OR/1
  Bitwise OR/1 -> Switch/2
  [validationTime] -> Switch/1
  Switch/1 -> Delay/1, Bus Creator/2  "validationTime"
  EcuAppM_BufferedWakeupSource/1 -> [EcuAppM_BufferedWakeupSource], Bitwise OR/2
  Bus Selector1/3 -> [wakeupReaction]  "<wakeupReaction>"
  [EcuAppM_BufferedWakeupSource] -> Bitwise OR1/2
  [wakeupMask] -> Bitwise OR1/1
  Bitwise OR1/1 -> Switch1/2
  Switch1/1 -> Delay1/1, Bus Creator/3  "wakeupReaction"
  [wakeupReaction] -> Switch1/1
  Switch2/1 -> Delay2/1, Bus Creator/1  "wakeupMask"
  [wakeupMask] -> Switch2/1
  Bitwise OR2/1 -> Switch2/2
  [wakeupMask] -> Bitwise OR2/1
  [EcuAppM_BufferedWakeupSource] -> Bitwise OR2/2
  Bus Creator/1 -> EcuAppM_BufferedDataOutput/1  "EcuAppM_BufferedDataOutput"
  Delay2/1 -> Switch2/3
  Delay/1 -> Switch/3
  Delay1/1 -> Switch1/3
